simulink model "CANsim"  (Simulink 10.0)
settings: Solver=VariableStepAuto  StartTime=0.0  StopTime=10  RelTol=1e-3
undefined symbols (not defined in the file or in its folder): canChannel
libraries: canlib x5, canmsglib x4
settings Model: LogicAnalyzerSignalOrdering=19327169-cb2c-40fb-99c7-8bf09050f896,7e47515b-78e1-41c0-9481-691a97a6f306  Creator=krishna  LastModifiedBy=krishna  EnablePacing=on
settings DataIOCC: SaveFormat=Dataset  ReturnWorkspaceOutputs=on
settings OptimizationCC: LifeSpan=auto
settings DebuggingCC: UnderspecifiedInitializationDetection=Simplified  MergeDetectMultiDrivingBlocksExec=error  SFUnexpectedBacktrackingDiag=error  SFNoUnconditionalDefaultTransitionDiag=error  SFExecutionAtInitializationDiag=warning  ArithmeticOperatorsInVariantConditions=error
settings HardwareCC: ProdBitPerPointer=64  ProdBitPerSizeT=64  ProdBitPerPtrDiffT=64  ProdLargestAtomicFloat=Float  ProdIntDivRoundTo=Zero  ProdEndianess=LittleEndian  ProdWordSize=64  ProdHWDeviceType=Intel->x86-64 (Windows64)
settings ModelReferenceCC: PropagateSignalLabelsOutOfModel=on
settings SFSimCC: SimUseLocalCustomCode=on  CustomCodeUndefinedFunction=FilterOut
settings RTWCC: RTWUseLocalCustomCode=on
settings CodeAppCC: StateflowObjectComments=off
settings GRTTargetCC: TargetLangStandard=C99 (ISO)  CombineOutputUpdateFcns=on  GRTInterface=off
settings ConfigComp: CovMetricSettings=dwe  CovHtmlReporting=off  CovSaveCumulativeToWorkspaceVar=off  CovSaveSingleToWorkspaceVar=off

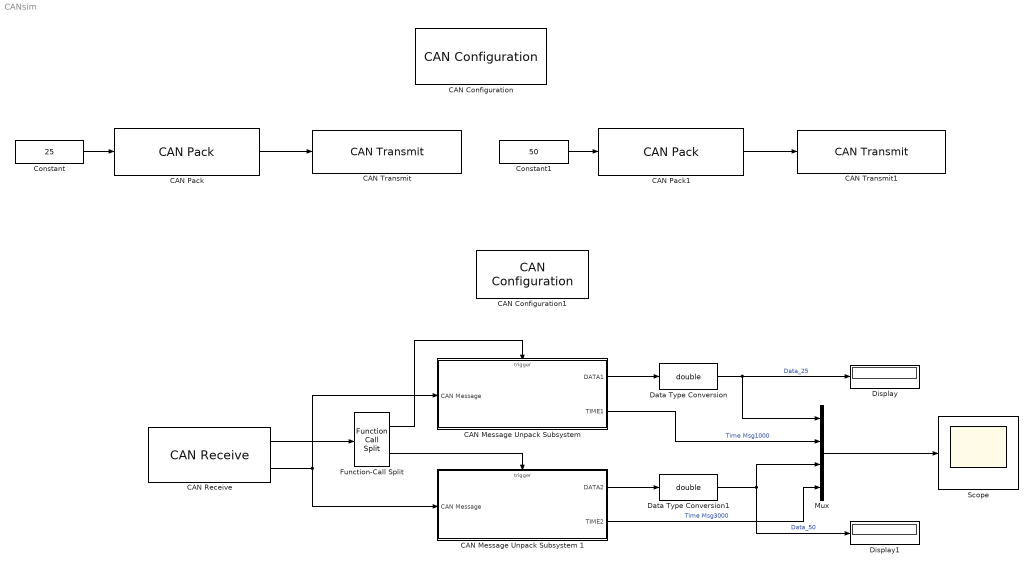
== system CANsim ==
  CAN Configuration : canlib/CAN Configuration  BlockHandle=5.0002  Device=MathWorks Virtual 1 (Channel 1)  DeviceMenu=MathWorks Virtual 1 (Channel 1)  ObjConstructor=canChannel('MathWorks', 'Virtual 1', 1)  BusSpeed=500000  EnableBitParameters=off  AckMode=Normal
      settings: SourceProductName=Vehicle Network Toolbox  SourceProductBaseCode=VN
  CAN Configuration1 : canlib/CAN Configuration  BlockHandle=5.0002  Device=MathWorks Virtual 1 (Channel 2)  DeviceMenu=MathWorks Virtual 1 (Channel 2)  ObjConstructor=canChannel('MathWorks', 'Virtual 1', 2)  BusSpeed=500000  EnableBitParameters=off  AckMode=Normal
      settings: SourceProductName=Vehicle Network Toolbox  SourceProductBaseCode=VN
  "CAN Message Unpack Subsystem " : Subsystem  TreatAsAtomicUnit=on
  CAN Message Unpack Subsystem 1 : Subsystem  TreatAsAtomicUnit=on
  CAN Pack : canmsglib/CAN Pack  MsgList=(none)  MsgName=CAN Msg  MsgIDType=Extended (29-bit identifier)  MsgIdentifier=1000  MsgLength=8  Remote=off  ApplyMinMax=off  BusOutput=off  SignalInfo={}
      settings: SourceProductName=Vehicle Network Toolbox  SourceProductBaseCode=VN  DataFormat=raw data
  CAN Pack1 : canmsglib/CAN Pack  MsgList=(none)  MsgName=CAN Msg  MsgIDType=Extended (29-bit identifier)  MsgIdentifier=3000  MsgLength=8  Remote=off  ApplyMinMax=off  BusOutput=off  SignalInfo={}
      settings: SourceProductName=Vehicle Network Toolbox  SourceProductBaseCode=VN  DataFormat=raw data
  CAN Receive : canlib/CAN Receive  BlockHandle=8.0002  Device=MathWorks Virtual 1 (Channel 2)  DeviceMenu=MathWorks Virtual 1 (Channel 2)  ObjConstructor=canChannel('MathWorks', 'Virtual 1', 2)  EnableStandardIDsFilter=off  StdIDsCombo=Allow all  StandardIDs=0  EnableExtendedIDsFilter=off  ExtIDsCombo=Allow all  ExtendedIDs=0  SampleTime=0.01  MsgsPerTimestep=all  InternalFilterUpdateStatus=on  BusOutput=off
      settings: SourceProductName=Vehicle Network Toolbox  SourceProductBaseCode=VN
  CAN Transmit : canlib/CAN Transmit  BlockHandle=10.0002  Device=MathWorks Virtual 1 (Channel 1)  DeviceMenu=MathWorks Virtual 1 (Channel 1)  ObjConstructor=canChannel('MathWorks', 'Virtual 1', 1)  EnablePeriodicTransmit=on  MessagePeriod=0.5
      settings: SourceProductName=Vehicle Network Toolbox  SourceProductBaseCode=VN
  CAN Transmit1 : canlib/CAN Transmit  BlockHandle=10.0002  Device=MathWorks Virtual 1 (Channel 1)  DeviceMenu=MathWorks Virtual 1 (Channel 1)  ObjConstructor=canChannel('MathWorks', 'Virtual 1', 1)  EnablePeriodicTransmit=on  MessagePeriod=0.5
      settings: SourceProductName=Vehicle Network Toolbox  SourceProductBaseCode=VN
  Constant : Constant  Value=25  OutDataTypeStr=uint8  SampleTime=0.01
  Constant1 : Constant  Value=50  OutDataTypeStr=uint8  SampleTime=0.01
  Data Type Conversion : DataTypeConversion  OutDataTypeStr=double
  Data Type Conversion1 : DataTypeConversion  OutDataTypeStr=double
  Display : Display
  Display1 : Display
  Function-Call Split : FunctionCallSplit  IconShape=distinctive  NumOutputPorts=2  OutputPortLayout=default
  Mux : Mux
  Scope : Scope
  wires:
  Constant/1 -> CAN Pack/1
  CAN Pack/1 -> CAN Transmit/1
  Constant1/1 -> CAN Pack1/1
  CAN Pack1/1 -> CAN Transmit1/1
  CAN Receive/1 -> Function-Call Split/1
  Function-Call Split/1 -> "CAN Message Unpack Subsystem "/Trigger
  Function-Call Split/2 -> CAN Message Unpack Subsystem 1/Trigger
  CAN Receive/2 -> CAN Message Unpack Subsystem 1/1(CAN Message), "CAN Message Unpack Subsystem "/1(CAN Message)
  "CAN Message Unpack Subsystem "/1(DATA1) -> Data Type Conversion/1
  "CAN Message Unpack Subsystem "/2(TIME1) -> Mux/2  "Time Msg1000"
  CAN Message Unpack Subsystem 1/1(DATA2) -> Data Type Conversion1/1
  CAN Message Unpack Subsystem 1/2(TIME2) -> Mux/4  "Time Msg3000"
  Data Type Conversion/1 -> Mux/1, Display/1  "Data_25"
  Data Type Conversion1/1 -> Display1/1, Mux/3  "Data_50"
  Mux/1 -> Scope/1

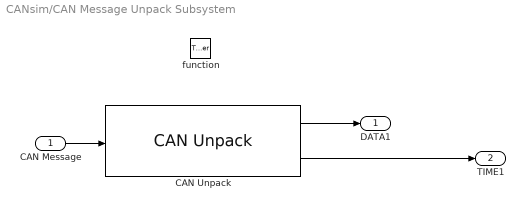
== system CANsim/CAN Message Unpack Subsystem  ==
  CAN Message : Inport
  function : TriggerPort  TriggerType=function-call  VariantControl=Variant
  CAN Unpack : canmsglib/CAN Unpack  MsgList=(none)  MsgName=CAN Msg  MsgIDType=Extended (29-bit identifier)  MsgIdentifier=1000  MsgLength=8  SignalInfo={}  IDPort=off  TimestampPort=on  ErrorPort=off  RemotePort=off  LengthPort=off  StatusPort=off  ApplyMinMax=off
      settings: SourceProductName=Vehicle Network Toolbox  SourceProductBaseCode=VN  DataFormat=raw data
  DATA1 : Outport
  TIME1 : Outport  Port=2
  wires:
  CAN Message/1 -> CAN Unpack/1
  CAN Unpack/1 -> DATA1/1
  CAN Unpack/2 -> TIME1/1

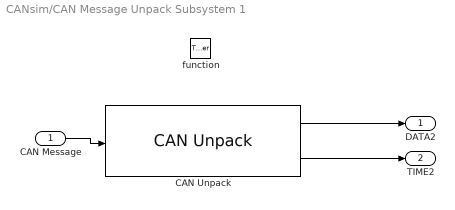
== system CANsim/CAN Message Unpack Subsystem 1 ==
  CAN Message : Inport
  function : TriggerPort  TriggerType=function-call  VariantControl=Variant
  CAN Unpack : canmsglib/CAN Unpack  MsgList=(none)  MsgName=CAN Msg  MsgIDType=Extended (29-bit identifier)  MsgIdentifier=3000  MsgLength=8  SignalInfo={}  IDPort=off  TimestampPort=on  ErrorPort=off  RemotePort=off  LengthPort=off  StatusPort=off  ApplyMinMax=off
      settings: SourceProductName=Vehicle Network Toolbox  SourceProductBaseCode=VN  DataFormat=raw data
  DATA2 : Outport
  TIME2 : Outport  Port=2
  wires:
  CAN Message/1 -> CAN Unpack/1
  CAN Unpack/1 -> DATA2/1
  CAN Unpack/2 -> TIME2/1
